simulink model "parte07"  (R2020b)
settings: Solver=VariableStepAuto  StartTime=0.0  StopTime=0.8  RelTol=1e-3
values from neighbouring files (symbols this model uses):
  A1 = [0,1,0; 0,0,1; -a0,-a1,-a2]    [Lab3.m]    (also in parte1.m)
  A2 = [ -a2,1,0;     -a1,0,1;     -a0,0,0]    [Lab3.m]    (also in parte1.m = [ -a0,1,0; -a1,0,1; -a0,0,-a2])
  A3 = [(-1*(r1+r2)/(r1*r2*c1)), (1/(r2*c1)), -1/(r2*c1); 0,0, -1/(r3*c2); -1/(r2*c3),1/(r2*c3), -1*(r2+r3)/(r2*r3*c3)]    [Lab3.m]    (also in parte1.m)
  A5 = linsys1.A    [Lab3.m]    (also in parte1.m = LinearAnalysisToolProject.LocalVariables.Value.A)
  B1 = [0; 0; 1]    [Lab3.m]    (also in parte1.m)
  B2 = [0; 0; b0]    [Lab3.m]    (also in parte1.m)
  B3 = [1/(r1*c1);0;0]    [Lab3.m]    (also in parte1.m)
  B5 = linsys1.B    [Lab3.m]    (also in parte1.m = LinearAnalysisToolProject.LocalVariables.Value.B)
  C1 = [b0,0,0]    [Lab3.m]    (also in parte1.m)
  C2 = [1,0,0]    [Lab3.m]    (also in parte1.m = [0,0,1])
  C3 = [0,1,0]    [Lab3.m]    (also in parte1.m)
  C5 = linsys1.C    [Lab3.m]    (also in parte1.m = LinearAnalysisToolProject.LocalVariables.Value.c)
  G0 = tf([b0], [1, a2, a1, a0])    [Lab3.m]    (also in parte1.m)
undefined symbols (not defined in the file or in its folder): A4, B4, C4
settings Model: Creator=julit  LastModifiedBy=julit

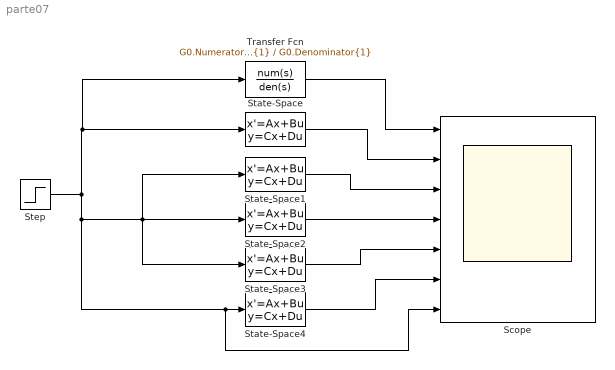
== system parte07 ==
  Scope : Scope  NumInputPorts=7
  State-Space : StateSpace  A=A1  B=B1  C=C1  D=0  InitialCondition=0
  State-Space1 : StateSpace  A=A2  B=B2  C=C2  D=0  InitialCondition=0
  State-Space2 : StateSpace  A=A3  B=B3  C=C3  D=0  InitialCondition=0
  State-Space3 : StateSpace  A=A4  B=B4  C=C4  D=0  InitialCondition=0
  State-Space4 : StateSpace  A=A5  B=B5  C=C5  D=0  InitialCondition=0
  Step : Step  Time=0.01  After=5  SampleTime=0.001
  Transfer Fcn : TransferFcn  Numerator=G0.Numerator{1}  Denominator=G0.Denominator{1}
  wires:
  Step/1 -> Scope/7, State-Space4/1, State-Space3/1, State-Space1/1, State-Space2/1, Transfer Fcn/1, State-Space/1
  Transfer Fcn/1 -> Scope/1
  State-Space/1 -> Scope/2
  State-Space1/1 -> Scope/3
  State-Space2/1 -> Scope/4
  State-Space3/1 -> Scope/5
  State-Space4/1 -> Scope/6
